simulink model "Engine"  (R2025a)
settings: Solver=VariableStepAuto  StartTime=0.0  StopTime=100  RelTol=1e-3
values from neighbouring files (symbols this model uses):
  Cm = 1.3    [activation.m]
  Cw = 3.15    [activation.m]
  Jdv = 7e-6    (= 7e-06)    [activation.m]
  Lj = 0.0015    [activation.m]
  Lov = 0.013    [activation.m]
  Rj = 8    [activation.m]
libraries: SignalEditorBlockLib x1
settings Model: Creator=Reymond  LastModifiedBy=Reymond

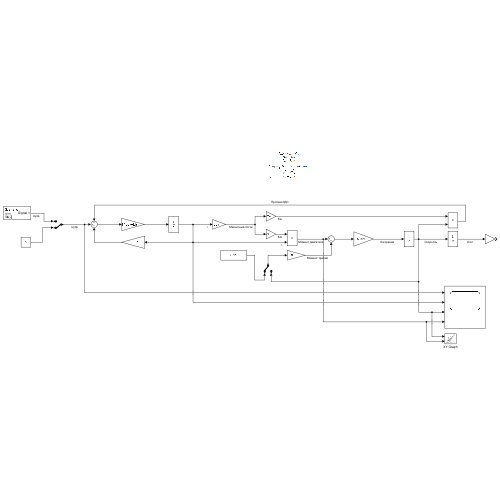
[thumbnail: Simulink's stored preview of the top-level diagram]
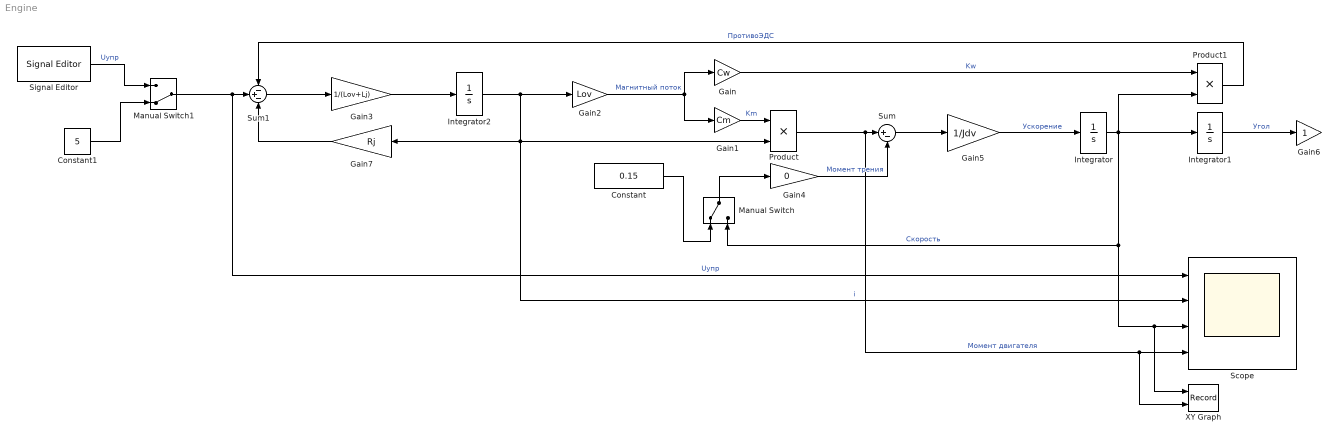
== system Engine ==
  Constant : Constant  Value=0.15
  Constant1 : Constant  Value=5
  Gain : Gain  Gain=Cw
  Gain1 : Gain  Gain=Cm
  Gain2 : Gain  Gain=Lov
  Gain3 : Gain  Gain=1/(Lov+Lj)
  Gain4 : Gain  Gain=0
  Gain5 : Gain  Gain=1/Jdv
  Gain6 : Gain
  Gain7 : Gain  Gain=Rj
  Integrator : Integrator
  Integrator1 : Integrator
  Integrator2 : Integrator
  Manual Switch : ManualSwitch
  Manual Switch1 : ManualSwitch  CurrentSetting=0
  Product : Product
  Product1 : Product
  Scope : Scope  NumInputPorts=4
      settings: ActiveDisplayString=4  ActiveDisplayYMinimum=-0.00017064896090497462  ActiveDisplayYMaximum=0.0015358406481447719
  Signal Editor : SignalEditorBlockLib/Signal Editor  FileName=signal.mat  ActiveScenario=Scenario  ActiveSignal=Signal 1  IsBus=off  OutputBusObjectStr=Bus: BusObject  SampleTime=0  ZeroCross=off  OutputAfterFinalValue=Setting to zero  Unit=inherit  PreserveSignalName=on  ApplySigPropsToAllScenarios=on  ApplySigPropsToAllSignals=off  SignalPropertySource=Dialog parameters
  Sum : Sum  Inputs=|+-
  Sum1 : Sum  Inputs=-+-
  XY Graph : Record  NumPorts=2.0  FileSettingsInternal="{\"entries\":[{\"content\":{\"excelSettings\":{\"content\":{},\"type\":\"Streamout.ExcelSettings\"},\"parquetSettings\":{\"content\":{},\"type\":\"Streamout.ParquetSettings\"}},\"type\":\"Streamout.FileSettingStorage\",\"uuid\":\"\"}],\"packageUris\":[\"http:\\/\\/schema.mathworks.com\\/mf0\\/streamout_blocks\\/R2020a\"],\"version\":\"1.0\"}"  FrameSettings=[0, 0]  Layout=[1 1]  SignalsInternal="{\"entries\":[{\"content\":{\"signals\":[{\"content\":{\"blockPath\":[],\"dimensions\":[1],\"domain\":\"\",\"lineColor\":\"#a2142f\",\"plots\":[ 1 ],\"port\":1,\"sid\":[\"\"],\"signalID\":1,\"signalName\":\"Скорость\"},\"type\":\"RecordBlkView.Signal\",\"uuid\":\"\"},{\"content\":{\"blockPath\":[],\"dimensions\":[1],\"domain\":\"\",\"lineColor\":\"#139fff\",\"plots\":[ 1 ],\"port\":2,\"sid\":[\"\"],\"signalID\":2,\"signalName\":\"Момент двигателя\"},\"type\":\"RecordBlkView.Signal\",\"uuid\":\"\"}]},\"type\":\"RecordBlkView.InputSignals\",\"uuid\":\"\"}],\"packageUris\":[\"http:\\/\\/schema.mathworks.com\\/mf0\\/streamout_blocks\\/R2020a\"],\"version\":\"1.0\"}"  VisualizationBindings="{\"xyplotplugin\":{\"info\":[{\"series\":[{\"bindingParametersList\":[{\"parameter\":\"X-Axis\",\"signalID\":1,\"signalName\":\"Скорость\"},{\"parameter\":\"Y-Axis\",\"signalID\":2,\"signalName\":\"Момент двигателя\"}],\"seriesID\":0}],\"subplotID\":1}]}}"  CompatibilityTag=XY
  wires:
  Gain2/1 -> Gain/1, Gain1/1  "Магнитный поток"
  Integrator2/1 -> Scope/2, Gain7/1, Product/2, Gain2/1  "i"
  Gain1/1 -> Product/1  "Km"
  Product/1 -> XY Graph/2, Scope/4, Sum/1  "Момент двигателя"
  Gain4/1 -> Sum/2  "Момент трения"
  Sum/1 -> Gain5/1
  Gain5/1 -> Integrator/1  "Ускорение"
  Integrator/1 -> XY Graph/1, Scope/3, Manual Switch/2, Product1/2, Integrator1/1  "Скорость"
  Integrator1/1 -> Gain6/1  "Угол"
  Gain/1 -> Product1/1  "Kw"
  Signal Editor/1 -> Manual Switch1/1  "Uупр"
  Sum1/1 -> Gain3/1
  Gain3/1 -> Integrator2/1
  Gain7/1 -> Sum1/3
  Product1/1 -> Sum1/1  "ПротивоЭДС"
  Constant/1 -> Manual Switch/1
  Manual Switch/1 -> Gain4/1
  Manual Switch1/1 -> Scope/1, Sum1/2  "Uупр"
  Constant1/1 -> Manual Switch1/2
